simulink library "Traffic_2_UL"  (R2020a)
settings: Solver=VariableStepAuto  StartTime=0.0  StopTime=10.0  RelTol=1e-3
undefined symbols (not defined in the file): DiscIntNeverNeededParam, Int, sig_info, stopping_profile, T_mode, t_start, Traffic
libraries: simulink x8
settings Model: Creator=John Jr  LastModifiedBy=John Jr
settings DataIOCC: ReturnWorkspaceOutputs=off
settings DebuggingCC: ArithmeticOperatorsInVariantConditions=warning
settings SFSimCC: CustomCodeUndefinedFunction=UseInterfaceOnly

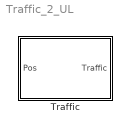
== system Traffic_2_UL ==
  Traffic : Subsystem
      mask Display:
      | patch([0 1 1 0], [0 0 1 1],[.8 1 1])
      | 
      | port_label('input',1,'Pos')
      | 
      | port_label('output',1,'Traffic')

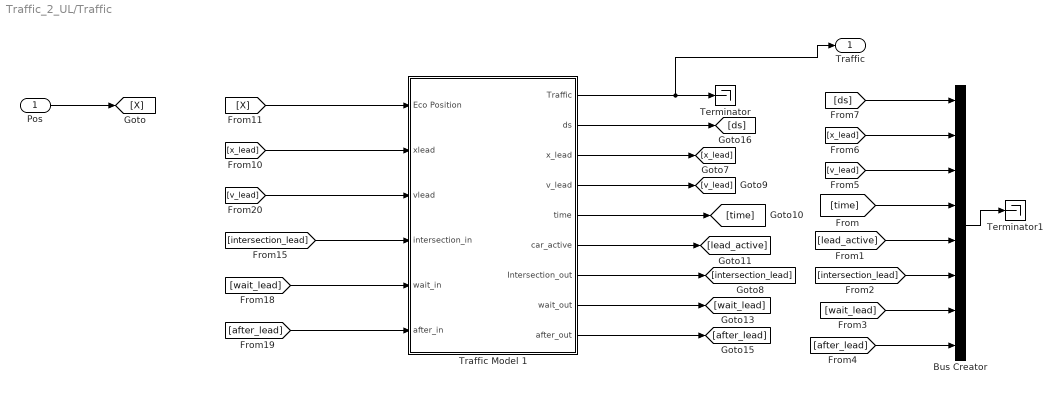
== system Traffic_2_UL/Traffic ==
  Pos : Inport
  Bus Creator : BusCreator  Inputs=8
  Terminator : Terminator
  Terminator1 : Terminator
  Traffic Model 1 : Subsystem
  Traffic : Outport  VectorParamsAs1DForOutWhenUnconnected=off
  wires:
  [ds] -> Bus Creator/1
  [x_lead] -> Bus Creator/2
  [v_lead] -> Bus Creator/3
  [time] -> Bus Creator/4
  [lead_active] -> Bus Creator/5
  [intersection_lead] -> Bus Creator/6
  [wait_lead] -> Bus Creator/7
  [after_lead] -> Bus Creator/8
  Traffic Model 1/3(x_lead) -> [x_lead]
  Traffic Model 1/6(car_active) -> [lead_active]
  [x_lead] -> Traffic Model 1/2(xlead)
  Traffic Model 1/4(v_lead) -> [v_lead]
  Traffic Model 1/9(after_out) -> [after_lead]
  [X] -> Traffic Model 1/1(Eco Position)
  Traffic Model 1/5(time) -> [time]
  Pos/1 -> [X]
  [after_lead] -> Traffic Model 1/6(after_in)
  Traffic Model 1/7(Intersection_out) -> [intersection_lead]
  [intersection_lead] -> Traffic Model 1/4(intersection_in)
  Traffic Model 1/2(ds) -> [ds]
  [v_lead] -> Traffic Model 1/3(vlead)
  Traffic Model 1/8(wait_out) -> [wait_lead]
  [wait_lead] -> Traffic Model 1/5(wait_in)
  Traffic Model 1/1(Traffic) -> Terminator/1, Traffic/1
  Bus Creator/1 -> Terminator1/1

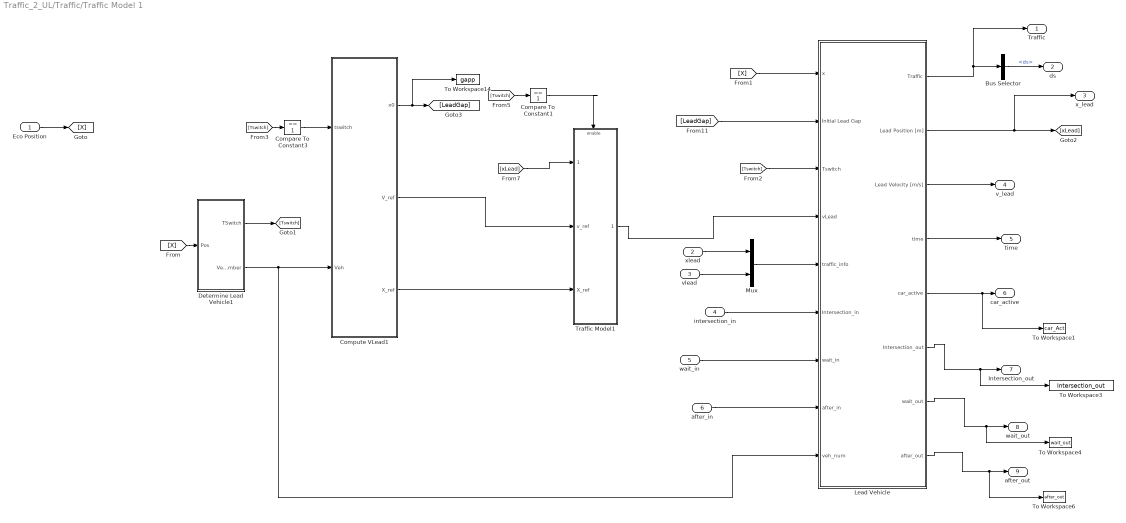
== system Traffic_2_UL/Traffic/Traffic Model 1 ==
  Eco Position : Inport
  xlead : Inport  Port=2
  vlead : Inport  Port=3
  intersection_in : Inport  Port=4
  wait_in : Inport  Port=5
  after_in : Inport  Port=6
  Bus Selector : BusSelector  OutputSignals=ds
  Compare To Constant1 : simulink/Logic and Bit Operations/Compare To Constant  relop===  const=1  OutDataTypeStr=boolean
  Compare To Constant3 : simulink/Logic and Bit Operations/Compare To Constant  relop===  const=1  OutDataTypeStr=boolean
  Compute VLead1 : Subsystem
  Determine Lead Vehicle1 : Subsystem
  Lead Vehicle : Subsystem
      settings: MinAlgLoopOccurrences=on
  Mux : Mux  Inputs=2
  To Workspace1 : ToWorkspace  VariableName=car_Act  SampleTime=.01
  To Workspace14 : ToWorkspace  VariableName=gapp  SampleTime=.01
  To Workspace3 : ToWorkspace  VariableName=Intersection_out  SampleTime=-1
  To Workspace4 : ToWorkspace  VariableName=wait_out  SampleTime=-1
  To Workspace6 : ToWorkspace  VariableName=after_out  SampleTime=-1
  Traffic Model1 : Subsystem
  Traffic : Outport  VectorParamsAs1DForOutWhenUnconnected=off
  ds : Outport  Port=2  VectorParamsAs1DForOutWhenUnconnected=off
  x_lead : Outport  Port=3  VectorParamsAs1DForOutWhenUnconnected=off
  v_lead : Outport  Port=4  VectorParamsAs1DForOutWhenUnconnected=off
  time : Outport  Port=5  VectorParamsAs1DForOutWhenUnconnected=off
  car_active : Outport  Port=6  VectorParamsAs1DForOutWhenUnconnected=off
  Intersection_out : Outport  Port=7  VectorParamsAs1DForOutWhenUnconnected=off
  wait_out : Outport  Port=8  VectorParamsAs1DForOutWhenUnconnected=off
  after_out : Outport  Port=9  VectorParamsAs1DForOutWhenUnconnected=off
  wires:
  Lead Vehicle/2(Lead Position [m]) -> [xLead], x_lead/1
  vlead/1 -> Mux/2
  [xLead] -> Traffic Model1/1(x_Lead)
  xlead/1 -> Mux/1
  Mux/1 -> Lead Vehicle/5(traffic_info)
  Bus Selector/1 -> ds/1  "<ds>"
  Traffic Model1/1(v_lead) -> Lead Vehicle/4(vLead)
  Compare To Constant1/1 -> Traffic Model1/Enable
  Determine Lead Vehicle1/2(Veh Number) -> Lead Vehicle/9(veh_num), Compute VLead1/2(Veh)
  intersection_in/1 -> Lead Vehicle/6(Intersection_in)
  wait_in/1 -> Lead Vehicle/7(wait_in)
  after_in/1 -> Lead Vehicle/8(after_in)
  Lead Vehicle/8(after_out) -> after_out/1, To Workspace6/1
  Lead Vehicle/7(wait_out) -> wait_out/1, To Workspace4/1
  Lead Vehicle/6(Intersection_out) -> Intersection_out/1, To Workspace3/1
  Lead Vehicle/5(car_active) -> car_active/1, To Workspace1/1
  Lead Vehicle/4(time) -> time/1
  Lead Vehicle/3(Lead Velocity [m/s]) -> v_lead/1
  Compute VLead1/3(X_ref) -> Traffic Model1/3(X_ref)
  Lead Vehicle/1(Traffic) -> Traffic/1, Bus Selector/1
  [Tswitch] -> Lead Vehicle/3(Tswitch)
  [X] -> Lead Vehicle/1(x)
  [LeadGap] -> Lead Vehicle/2(Initial Lead Gap)
  Compute VLead1/1(x0) -> [LeadGap], To Workspace14/1
  [Tswitch] -> Compare To Constant3/1
  Compute VLead1/2(V_ref) -> Traffic Model1/2(v_ref)
  Compare To Constant3/1 -> Compute VLead1/1(tswitch)
  [Tswitch] -> Compare To Constant1/1
  Determine Lead Vehicle1/1(TSwitch) -> [Tswitch]
  [X] -> Determine Lead Vehicle1/1(Pos)
  Eco Position/1 -> [X]

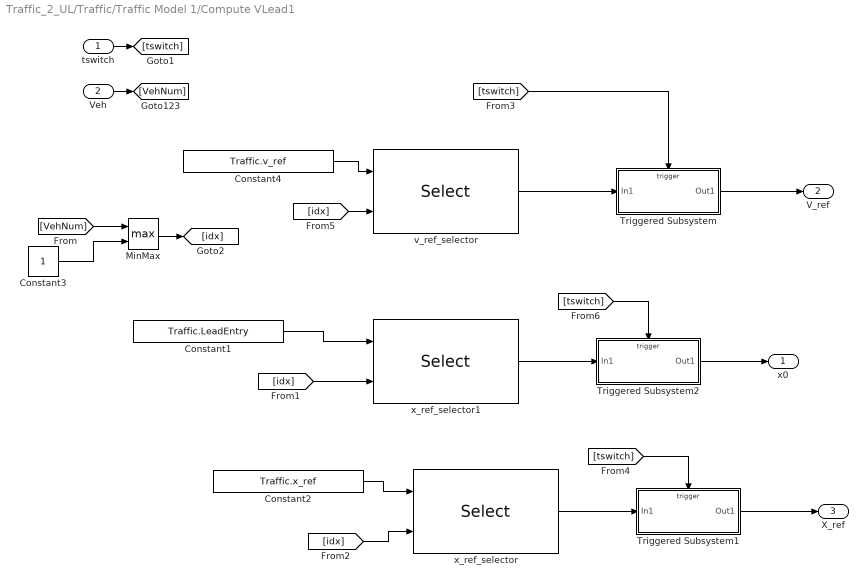
== system Traffic_2_UL/Traffic/Traffic Model 1/Compute VLead1 ==
  tswitch : Inport  PortDimensions=1
  Veh : Inport  Port=2  PortDimensions=1
  Constant1 : Constant  Value=Traffic.LeadEntry
  Constant2 : Constant  Value=Traffic.x_ref
  Constant3 : Constant
  Constant4 : Constant  Value=Traffic.v_ref
  MinMax : MinMax  Function=max  Inputs=2  InputSameDT=on
  Triggered Subsystem : Subsystem  TreatAsAtomicUnit=on
  Triggered Subsystem1 : Subsystem  TreatAsAtomicUnit=on
  Triggered Subsystem2 : Subsystem  TreatAsAtomicUnit=on
  v_ref_selector : Selector  NumberOfDimensions=2  InputPortWidth=3  IndexOptions=Select all,Index vector (port)  Indices=[1 3],1  OutputSizes=1,1
  x_ref_selector : Selector  NumberOfDimensions=2  InputPortWidth=3  IndexOptions=Select all,Index vector (port)  Indices=[1 3],1  OutputSizes=1,1
  x_ref_selector1 : Selector  InputPortWidth=40  IndexOptions=Index vector (port)  Indices=[1 3]  OutputSizes=1
  x0 : Outport  PortDimensions=1  VectorParamsAs1DForOutWhenUnconnected=off
  V_ref : Outport  Port=2  PortDimensions=[8000 1]  InitialOutput=ones(8000,1)  VectorParamsAs1DForOutWhenUnconnected=off
  X_ref : Outport  Port=3  PortDimensions=[8000 1]  VectorParamsAs1DForOutWhenUnconnected=off
  wires:
  [tswitch] -> Triggered Subsystem2/Trigger
  Triggered Subsystem2/1(Out1) -> x0/1
  x_ref_selector1/1 -> Triggered Subsystem2/1(In1)
  [idx] -> v_ref_selector/2
  [idx] -> x_ref_selector1/2
  Constant1/1 -> x_ref_selector1/1
  [tswitch] -> Triggered Subsystem1/Trigger
  Triggered Subsystem1/1(Out1) -> X_ref/1
  x_ref_selector/1 -> Triggered Subsystem1/1(In1)
  [idx] -> x_ref_selector/2
  MinMax/1 -> [idx]
  [tswitch] -> Triggered Subsystem/Trigger
  Triggered Subsystem/1(Out1) -> V_ref/1
  v_ref_selector/1 -> Triggered Subsystem/1(In1)
  tswitch/1 -> [tswitch]
  Constant3/1 -> MinMax/2
  [VehNum] -> MinMax/1
  Constant4/1 -> v_ref_selector/1
  Constant2/1 -> x_ref_selector/1
  Veh/1 -> [VehNum]

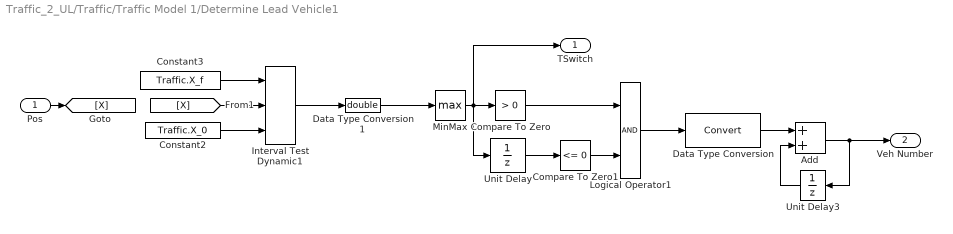
== system Traffic_2_UL/Traffic/Traffic Model 1/Determine Lead Vehicle1 ==
  Pos : Inport
  Add : Sum
  Compare To Zero : simulink/Logic and Bit Operations/Compare To Zero  relop=>  OutDataTypeStr=boolean
  Compare To Zero1 : simulink/Logic and Bit Operations/Compare To Zero  relop=<=  OutDataTypeStr=boolean
  Constant2 : Constant  Value=Traffic.X_0
  Constant3 : Constant  Value=Traffic.X_f
  Data Type Conversion : DataTypeConversion
  Data Type Conversion1 : DataTypeConversion  OutDataTypeStr=double
  Interval Test Dynamic1 : simulink/Logic and Bit Operations/Interval Test Dynamic  IntervalClosedRight=on  IntervalClosedLeft=on  OutDataTypeStr=boolean
      settings: SourceProductBaseCode=SL
  Logical Operator1 : Logic  OutDataTypeStr=boolean
  MinMax : MinMax  Function=max
  Unit Delay : UnitDelay  SampleTime=-1  HasFrameUpgradeWarning=on
  Unit Delay3 : UnitDelay  SampleTime=-1  HasFrameUpgradeWarning=on
  TSwitch : Outport  VectorParamsAs1DForOutWhenUnconnected=off
  Veh Number : Outport  Port=2  VectorParamsAs1DForOutWhenUnconnected=off
  wires:
  Pos/1 -> [X]
  [X] -> Interval Test Dynamic1/2
  Constant3/1 -> Interval Test Dynamic1/1
  Constant2/1 -> Interval Test Dynamic1/3
  Interval Test Dynamic1/1 -> Data Type Conversion1/1
  MinMax/1 -> TSwitch/1, Unit Delay/1, Compare To Zero/1
  Unit Delay/1 -> Compare To Zero1/1
  Compare To Zero1/1 -> Logical Operator1/2
  Compare To Zero/1 -> Logical Operator1/1
  Unit Delay3/1 -> Add/2
  Add/1 -> Veh Number/1, Unit Delay3/1
  Logical Operator1/1 -> Data Type Conversion/1
  Data Type Conversion/1 -> Add/1
  Data Type Conversion1/1 -> MinMax/1

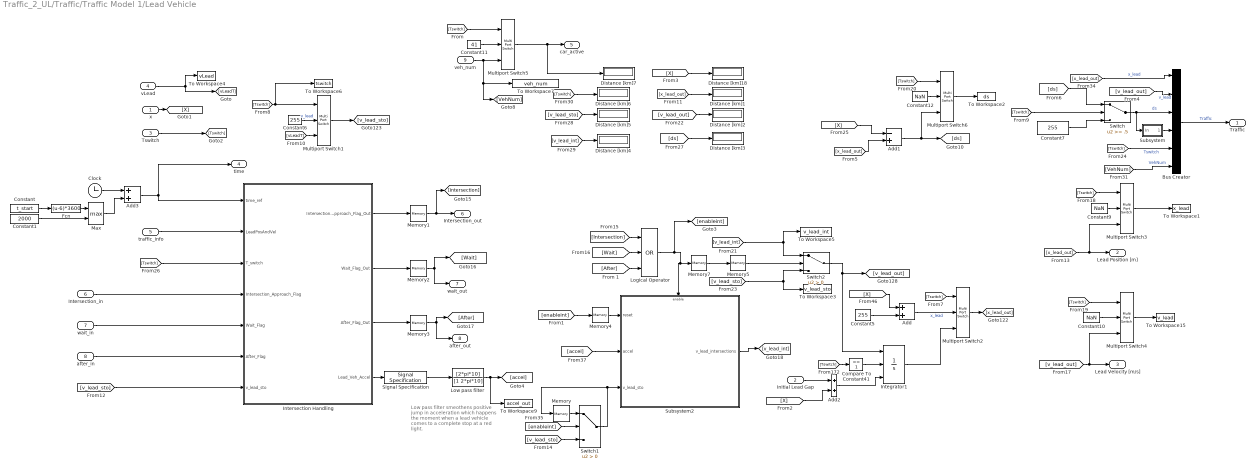
== system Traffic_2_UL/Traffic/Traffic Model 1/Lead Vehicle ==
  note: Low pass filter smeothens
      | positive jump in acceleration which
      | happens the moment when a lead
      | vehicle comes to a complete stop
      | at a red light.
  x : Inport
  Initial Lead Gap : Inport  Port=2
  Tswitch : Inport  Port=3
  vLead : Inport  Port=4
  traffic_info : Inport  Port=5
  Intersection_in : Inport  Port=6
  wait_in : Inport  Port=7
  after_in : Inport  Port=8
  veh_num : Inport  Port=9
  Add : Sum
  Add1 : Sum  Inputs=-+
  Add2 : Sum
  Add3 : Sum
  Bus Creator : BusCreator  Inputs=6
  Clock : Clock
      settings: Decimation=100
  Compare To Constant41 : simulink/Logic and Bit Operations/Compare To Constant  relop===  const=1  OutDataTypeStr=boolean
  Constant : Constant  Value=t_start
  Constant1 : Constant  Value=2000
  Constant10 : Constant  Value=NaN
  Constant11 : Constant  Value=41
  Constant12 : Constant  Value=NaN
  Constant5 : Constant  Value=255
  Constant6 : Constant  Value=255
  Constant7 : Constant  Value=255
  Constant9 : Constant  Value=NaN
  Distance [km]{1..7,18} (8 alike) : Display
      settings: Format=bank  Decimation=2
  Fcn : Fcn  Expr=(u-6)*3600
  Integrator1 : Integrator  ExternalReset=rising  InitialConditionSource=external  InitialCondition=2050  LimitOutput=on  LowerSaturationLimit=0
  Intersection Handling : Subsystem
  Logical Operator : Logic  Operator=OR  Inputs=3  AllPortsSameDT=off  OutDataTypeStr=boolean
  Low pass filter : TransferFcn  Numerator=[2*pi*10]  Denominator=[1 2*pi*10]
  Max : MinMax  Function=max  Inputs=2
  Memory{,1..5,7} (7 alike) : Memory
  Multiport Switch{1..6} (6 alike) : MultiPortSwitch  DataPortOrder=Zero-based contiguous  Inputs=2  DiagnosticForDefault=None  zeroidx=on
  Signal Specification : SignalSpecification  Dimensions=1
  Subsystem : Subsystem
  Subsystem2 : Subsystem
  Switch : Switch  Threshold=.5
  Switch1 : Switch  Criteria=u2 > Threshold
  Switch2 : Switch  Criteria=u2 > Threshold
  To Workspace1 : ToWorkspace  VariableName=x_lead  SampleTime=-1
  To Workspace15 : ToWorkspace  VariableName=v_lead  SampleTime=-1
  To Workspace2 : ToWorkspace  VariableName=ds  SampleTime=-1
  To Workspace3 : ToWorkspace  VariableName=v_lead_sto  SampleTime=-1
  To Workspace4 : ToWorkspace  VariableName=vLead  SampleTime=-1
  To Workspace5 : ToWorkspace  VariableName=v_lead_int  SampleTime=-1
  To Workspace6 : ToWorkspace  VariableName=tswitch  SampleTime=-1
  To Workspace7 : ToWorkspace  VariableName=veh_num  SampleTime=-1
  To Workspace9 : ToWorkspace  VariableName=accel_out  SampleTime=-1
  Traffic : Outport  VectorParamsAs1DForOutWhenUnconnected=off
  Lead Position [m] : Outport  Port=2  VectorParamsAs1DForOutWhenUnconnected=off
  Lead Velocity [m/s] : Outport  Port=3  VectorParamsAs1DForOutWhenUnconnected=off
  time : Outport  Port=4  VectorParamsAs1DForOutWhenUnconnected=off
  car_active : Outport  Port=5  VectorParamsAs1DForOutWhenUnconnected=off
  Intersection_out : Outport  Port=6  VectorParamsAs1DForOutWhenUnconnected=off
  wait_out : Outport  Port=7  VectorParamsAs1DForOutWhenUnconnected=off
  after_out : Outport  Port=8  VectorParamsAs1DForOutWhenUnconnected=off
  wires:
  Memory5/1 -> Switch2/2
  Memory4/1 -> Subsystem2/1("reset ")
  [enableint] -> Memory4/1
  Memory7/1 -> Memory5/1
  [v_lead_sto] -> Switch1/3
  [enableint] -> Switch1/2
  Memory/1 -> Switch1/1
  Low pass filter/1 -> [accel], To Workspace9/1
  Signal Specification/1 -> Low pass filter/1
  Switch1/1 -> Subsystem2/3("v_lead_sto "), Memory/1
  Intersection Handling/4(Lead_Veh_Accel) -> Signal Specification/1
  [Tswitch] -> Distance [km]6/1
  [v_lead_sto] -> Distance [km]5/1
  [v_lead_int] -> Distance [km]4/1
  [ds] -> Distance [km]3/1
  [v_lead_out] -> Distance [km]2/1
  [x_lead_out] -> Distance [km]1/1
  [X] -> Distance [km]18/1
  Memory3/1 -> after_out/1, [After]
  Memory2/1 -> [Wait], wait_out/1
  Memory1/1 -> Intersection_out/1, [Intersection]
  Intersection Handling/2(Wait_Flag_Out) -> Memory2/1
  Intersection Handling/3(After_Flag_Out) -> Memory3/1
  [Intersection] -> Logical Operator/1
  [Wait] -> Logical Operator/2
  [After] -> Logical Operator/3
  [v_lead_sto] -> Intersection Handling/7(v_lead_sto)
  after_in/1 -> Intersection Handling/6(After_Flag)
  wait_in/1 -> Intersection Handling/5(Wait_Flag)
  Intersection_in/1 -> Intersection Handling/4(Intersection_Approach_Flag)
  [Tswitch] -> Intersection Handling/3(T_switch)
  traffic_info/1 -> Intersection Handling/2(LeadPosAndVel)
  Intersection Handling/1("Intersection_Approach_Flag_Out ") -> Memory1/1
  Add3/1 -> time/1, Intersection Handling/1(time_ref)
  Multiport Switch6/1 -> To Workspace2/1
  Constant12/1 -> Multiport Switch6/2
  Add1/1 -> [ds], Multiport Switch6/3
  [Tswitch] -> Multiport Switch6/1
  Multiport Switch4/1 -> To Workspace15/1
  Constant10/1 -> Multiport Switch4/2
  [v_lead_out] -> Lead Velocity [m/s]/1, Multiport Switch4/3
  [Tswitch] -> Multiport Switch4/1
  Multiport Switch3/1 -> To Workspace1/1
  [Tswitch] -> Multiport Switch3/1
  Constant9/1 -> Multiport Switch3/2
  [x_lead_out] -> Lead Position [m]/1, Multiport Switch3/3
  Switch2/1 -> [v_lead_out], Integrator1/1
  Subsystem2/1(v_lead_intersections) -> [v_lead_int]
  Logical Operator/1 -> Memory7/1, Subsystem2/Enable, [enableint]
  [v_lead_sto] -> To Workspace3/1, Switch2/3
  [v_lead_int] -> Switch2/1, To Workspace5/1
  [accel] -> Subsystem2/2(accel)
  Constant5/1 -> Add/2
  [X] -> Add/1
  [x_lead_out] -> Add1/2
  [X] -> Add1/1
  Tswitch/1 -> [Tswitch]
  Constant11/1 -> Multiport Switch5/2
  veh_num/1 -> Multiport Switch5/3, To Workspace7/1, [VehNum]
  Multiport Switch5/1 -> car_active/1, Distance [km]7/1
  [Tswitch] -> Multiport Switch5/1
  Bus Creator/1 -> Traffic/1  "Traffic"
  x/1 -> [X]
  [vLeadT] -> Multiport Switch1/3
  Constant6/1 -> Multiport Switch1/2  "v_lead"
  Multiport Switch1/1 -> [v_lead_sto]
  [Tswitch] -> Multiport Switch1/1, To Workspace6/1
  Integrator1/1 -> Multiport Switch2/3
  [Tswitch] -> Multiport Switch2/1
  Add/1 -> Multiport Switch2/2  "x_lead"
  [Tswitch] -> Compare To Constant41/1
  Multiport Switch2/1 -> [x_lead_out]
  [X] -> Add2/2
  Add2/1 -> Integrator1/3
  Compare To Constant41/1 -> Integrator1/2
  vLead/1 -> [vLeadT], To Workspace4/1
  Initial Lead Gap/1 -> Add2/1
  [x_lead_out] -> Bus Creator/1  "x_lead"
  Subsystem/1(out) -> Bus Creator/4
  [Tswitch] -> Bus Creator/5  "Tswitch"
  Switch/1 -> Subsystem/1(In), Bus Creator/3  "ds"
  [ds] -> Switch/1
  [v_lead_out] -> Bus Creator/2  "v_lead"
  [VehNum] -> Bus Creator/6  "VehNum"
  Constant7/1 -> Switch/3
  [Tswitch] -> Switch/2
  Constant/1 -> Fcn/1
  Clock/1 -> Add3/1
  Fcn/1 -> Max/1
  Constant1/1 -> Max/2
  Max/1 -> Add3/2

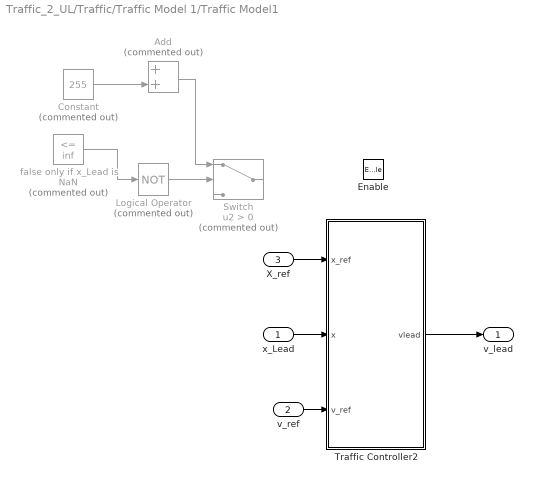
== system Traffic_2_UL/Traffic/Traffic Model 1/Traffic Model1 ==
  x_Lead : Inport
  v_ref : Inport  Port=2
  X_ref : Inport  Port=3
  Enable : EnablePort
  Add : Sum  Commented=on
  Constant : Constant  Commented=on  Value=255
  Logical Operator : Logic  Commented=on  Operator=NOT  AllPortsSameDT=off  OutDataTypeStr=boolean
  Switch : Switch  Commented=on  Criteria=u2 > Threshold
  Traffic Controller2 : MATLAB Function  TreatAsAtomicUnit=on
  false only if x_Lead is NaN : simulink/Logic and Bit Operations/Compare To Constant  Commented=on  relop=<=  const=inf  OutDataTypeStr=boolean
  v_lead : Outport  VectorParamsAs1DForOutWhenUnconnected=off
  wires:
  x_Lead/1 -> Traffic Controller2/2(x)
  Add/1 -> Switch/1
  Logical Operator/1 -> Switch/2
  Constant/1 -> Add/2
  false only if x_Lead is NaN/1 -> Logical Operator/1
  Traffic Controller2/1(vlead) -> v_lead/1
  v_ref/1 -> Traffic Controller2/3(v_ref)
  X_ref/1 -> Traffic Controller2/1(x_ref)

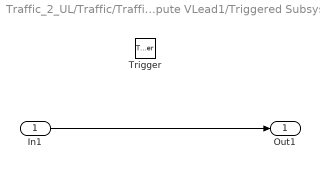
== system Traffic_2_UL/Traffic/Traffic Model 1/Compute VLead1/Triggered Subsystem ==
  In1 : Inport  PortDimensions=[8000 1]
  Trigger : TriggerPort  VariantControl=Variant
  Out1 : Outport  VectorParamsAs1DForOutWhenUnconnected=off
  wires:
  In1/1 -> Out1/1

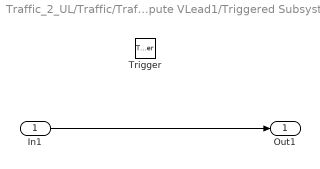
== system Traffic_2_UL/Traffic/Traffic Model 1/Compute VLead1/Triggered Subsystem1 ==
  In1 : Inport  PortDimensions=[8000 1]
  Trigger : TriggerPort  VariantControl=Variant
  Out1 : Outport  VectorParamsAs1DForOutWhenUnconnected=off
  wires:
  In1/1 -> Out1/1

== system Traffic_2_UL/Traffic/Traffic Model 1/Compute VLead1/Triggered Subsystem2 ==
  In1 : Inport  PortDimensions=1
  Trigger : TriggerPort  VariantControl=Variant
  Out1 : Outport  VectorParamsAs1DForOutWhenUnconnected=off
  wires:
  In1/1 -> Out1/1

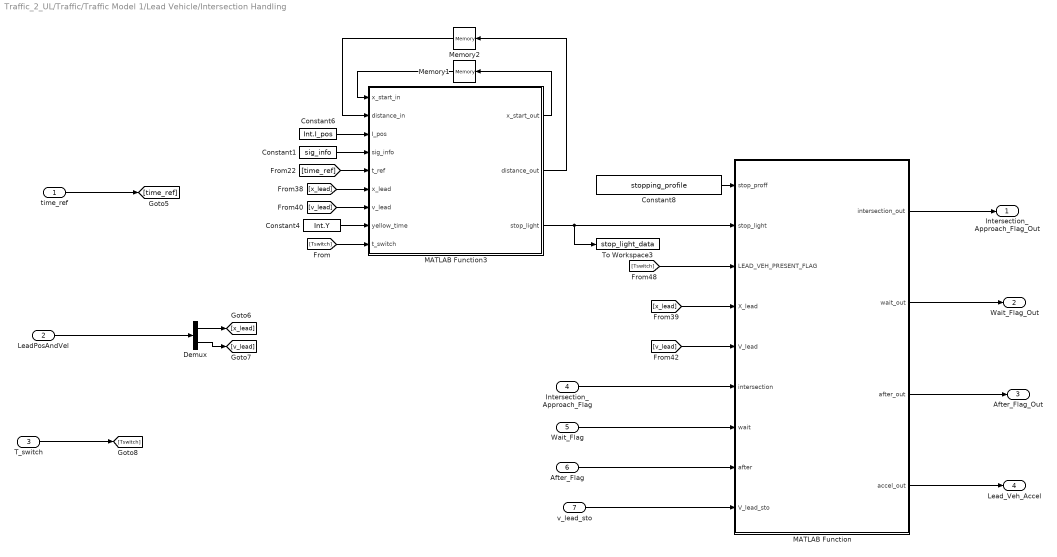
== system Traffic_2_UL/Traffic/Traffic Model 1/Lead Vehicle/Intersection Handling ==
  time_ref : Inport
  LeadPosAndVel : Inport  Port=2
  T_switch : Inport  Port=3
  Intersection_Approach_Flag : Inport  Port=4
  Wait_Flag : Inport  Port=5
  After_Flag : Inport  Port=6
  v_lead_sto : Inport  Port=7
  Constant1 : Constant  Value=sig_info
  Constant4 : Constant  Value=Int.Y
  Constant6 : Constant  Value=Int.I_pos
  Constant8 : Constant  Value=stopping_profile
  Demux : Demux  Outputs=2
  MATLAB Function : MATLAB Function  TreatAsAtomicUnit=on
  MATLAB Function3 : MATLAB Function  TreatAsAtomicUnit=on
  Memory1 : Memory
  Memory2 : Memory
  To Workspace3 : ToWorkspace  VariableName=stop_light_data  SampleTime=-1
  "Intersection_Approach_Flag_Out " : Outport  VectorParamsAs1DForOutWhenUnconnected=off
  Wait_Flag_Out : Outport  Port=2  VectorParamsAs1DForOutWhenUnconnected=off
  After_Flag_Out : Outport  Port=3  VectorParamsAs1DForOutWhenUnconnected=off
  Lead_Veh_Accel : Outport  Port=4  VectorParamsAs1DForOutWhenUnconnected=off
  wires:
  LeadPosAndVel/1 -> Demux/1
  [Tswitch] -> MATLAB Function3/9(t_switch)
  T_switch/1 -> [Tswitch]
  [time_ref] -> MATLAB Function3/5(t_ref)
  v_lead_sto/1 -> MATLAB Function/9(V_lead_sto)
  time_ref/1 -> [time_ref]
  [x_lead] -> MATLAB Function3/6(x_lead)
  [v_lead] -> MATLAB Function3/7(v_lead)
  Demux/2 -> [v_lead]
  Demux/1 -> [x_lead]
  [v_lead] -> MATLAB Function/5(V_lead)
  [x_lead] -> MATLAB Function/4(X_lead)
  [Tswitch] -> MATLAB Function/3(LEAD_VEH_PRESENT_FLAG)
  MATLAB Function/4(accel_out) -> Lead_Veh_Accel/1
  Wait_Flag/1 -> MATLAB Function/7(wait)
  After_Flag/1 -> MATLAB Function/8(after)
  MATLAB Function3/3(stop_light) -> MATLAB Function/2(stop_light), To Workspace3/1
  MATLAB Function3/1(x_start_out) -> Memory1/1
  MATLAB Function3/2(distance_out) -> Memory2/1
  MATLAB Function/1(intersection_out) -> "Intersection_Approach_Flag_Out "/1
  MATLAB Function/2(wait_out) -> Wait_Flag_Out/1
  Constant4/1 -> MATLAB Function3/8(yellow_time)
  Constant6/1 -> MATLAB Function3/3(I_pos)
  MATLAB Function/3(after_out) -> After_Flag_Out/1
  Intersection_Approach_Flag/1 -> MATLAB Function/6(intersection)
  Memory1/1 -> MATLAB Function3/1(x_start_in)
  Constant8/1 -> MATLAB Function/1(stop_proff)
  Memory2/1 -> MATLAB Function3/2(distance_in)
  Constant1/1 -> MATLAB Function3/4(sig_info)

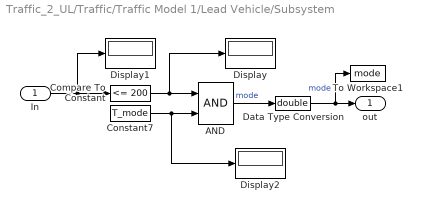
== system Traffic_2_UL/Traffic/Traffic Model 1/Lead Vehicle/Subsystem ==
  In : Inport
  AND : Logic  IconShape=distinctive  AllPortsSameDT=off  OutDataTypeStr=boolean
  Compare To Constant : simulink/Logic and Bit Operations/Compare To Constant  relop=<=  const=200  OutDataTypeStr=boolean
  Constant7 : Constant  Value=T_mode
  Data Type Conversion : DataTypeConversion  OutDataTypeStr=double
  Display : Display
  Display1 : Display
  Display2 : Display
  To Workspace1 : ToWorkspace  VariableName=mode  SampleTime=-1
  out : Outport  VectorParamsAs1DForOutWhenUnconnected=off
  wires:
  Constant7/1 -> Display2/1, AND/2
  Compare To Constant/1 -> Display/1, AND/1
  In/1 -> Display1/1, Compare To Constant/1
  AND/1 -> Data Type Conversion/1  "mode"
  Data Type Conversion/1 -> To Workspace1/1, out/1  "mode"

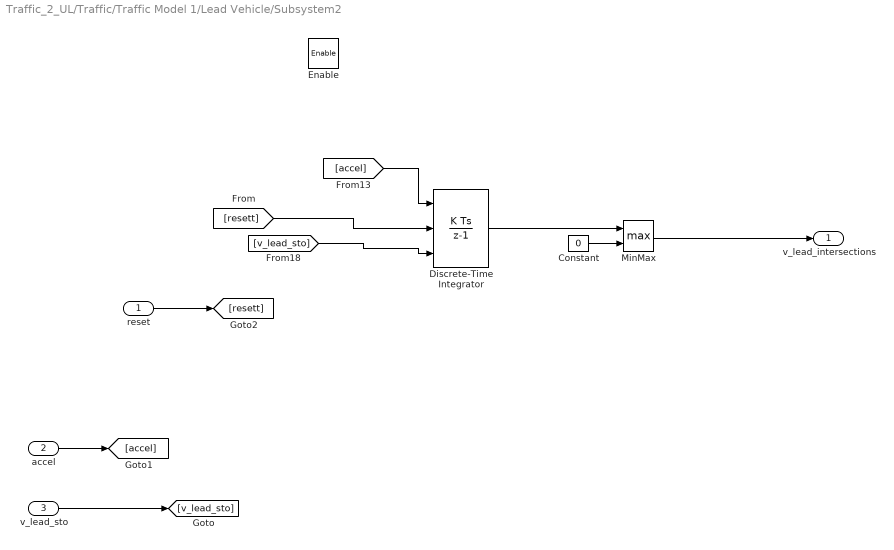
== system Traffic_2_UL/Traffic/Traffic Model 1/Lead Vehicle/Subsystem2 ==
  "reset " : Inport
  accel : Inport  Port=2
  "v_lead_sto " : Inport  Port=3
  Enable : EnablePort
  Constant : Constant  Value=0
  Discrete-Time Integrator : DiscreteIntegrator  ExternalReset=rising  InitialConditionSource=external  SampleTime=-1  ICPrevOutput=DiscIntNeverNeededParam  ICPrevScaledInput=DiscIntNeverNeededParam
  MinMax : MinMax  Function=max  Inputs=2
  v_lead_intersections : Outport  VectorParamsAs1DForOutWhenUnconnected=off
  wires:
  [resett] -> Discrete-Time Integrator/2
  "reset "/1 -> [resett]
  Constant/1 -> MinMax/2
  MinMax/1 -> v_lead_intersections/1
  "v_lead_sto "/1 -> [v_lead_sto]
  accel/1 -> [accel]
  [accel] -> Discrete-Time Integrator/1
  Discrete-Time Integrator/1 -> MinMax/1
  [v_lead_sto] -> Discrete-Time Integrator/3

== matlab function Traffic_2_UL/Traffic/Traffic Model 1/Lead Vehicle/Intersection Handling/MATLAB Function ==
  data: stop_proff input; stop_light input; LEAD_VEH_PRESENT_FLAG input; X_lead input; V_lead input; intersection input; wait input; after input; V_lead_sto input; intersection_out output; wait_out output; after_out output; accel_out output
function [intersection_out, wait_out, after_out,...
      accel_out] = intersection_sim(stop_proff, stop_light,...
      LEAD_VEH_PRESENT_FLAG, X_lead,V_lead, intersection, wait, after,...
      V_lead_sto)
% https://www.sciencedirect.com/science/article/pii/S1474667016442102   [1]
% http://ieeexplore.ieee.org/stamp/stamp.jsp?tp=&arnumber=6214590       [2]
lookahead_distance = 200;
stopping_profile = stop_proff;
buffer = 5;

if LEAD_VEH_PRESENT_FLAG == 0
    accel_out = 0;
    intersection_out = 0;
    wait_out = 0;
    after_out = 0;

else

    stop_location = stop_light(1);
    if intersection == 1   %Intersection flag has already been initialted
    %% approaching intersection
        if stop_location == 0 %light turns green during intersection approach phase
            after_out = 1;
            wait_out = 0;
            intersection_out = 0;
            accel_out = 0;
        else
            a_bstar = stopping_profile(3,:);
            x_bstar = stopping_profile(1,:);
            v_bstar = stopping_profile(2,:);
            X_q = -X_lead + (stop_location - buffer);
            v_bstar_val = interpone(x_bstar, v_bstar, X_q, 'str', 0);
            a_bstar_val = interpone(x_bstar, a_bstar, X_q, 'str', 0);
            accel = a_bstar_val*(V_lead/v_bstar_val)^2;       %   equation 9 of paper [2]

            if stop_location - X_lead < 0.02  %need to add a case for when if v_lead <0.1ms stop
                accel_out = 0;
                intersection_out = 0;
                wait_out = 1;
                after_out = 0;
            else
                accel_out = accel;
                intersection_out = 1;
                wait_out = 0;
                after_out = 0;
            end
        end
    elseif wait == 1   % wait_outing for light to turn green
    %% stopped at light
        if stop_location == 0 %  light turns green
            after_out = 1;
            wait_out = 0;
            intersection_out = 0;
            accel_out = 1;
        else
            accel_out = 1;
            intersection_out = 0;
            wait_out = 1;
            after_out = 0;
        end
    elseif after == 1       %   light has turned green
        %% leaving light after slowing down or stopping (intersection case entered beforehand)
        if V_lead_sto - V_lead <= 0.1 && V_lead_sto - V_lead >= -0.1 %reaches stochastic velocity
            intersection_out = 0;
            wait_out = 0;
            after_out = 0;
            accel_out = 0; % m/s^2
        elseif stop_location - X_lead < min(60*V_lead, lookahead_distance) && stop_location - X_lead > 0 %another intersection appears while accelerating to stochastic velocity profile.
            accel_out = 0;
            intersection_out = 1;
            wait_out = 0;
            after_out = 0;
        elseif V_lead_sto - V_lead > 0.1
            accel_out = 1; % m/s^2
            intersection_out = 0;
            wait_out = 0;
            after_out = 1;
        else
            accel_out = -1; % m/s^2   shouldn't happen
            intersection_out = 0;
            wait_out = 0;
            after_out = 1;
        end
    else
        if stop_location - X_lead < lookahead_distance && stop_location - X_lead > 0
            intersection_out = 1;
            wait_out = 0;
            after_out = 0;
            accel_out = 0;
        else
            accel_out = 0;
            intersection_out = 0;
            wait_out = 0;
            after_out = 0;
        end
    end
end
end
function return_val = interpone(X_data, Y_data, X_q, str, extrapval)
    if X_q >= X_data(1) && X_q <= X_data(end) 
        [~, I] = min((X_q - X_data).^2);
        if X_data(I) > X_q
            x_ub = X_data(I);
            x_lb = X_data(I-1);
            ind_xub = I;
            ind_xlb = I-1;
        else
            x_lb = X_data(I);
            ind_xlb = I;
            if I+1 >= length(X_data)    % M is probably equal to X_q and also the max value 
                x_lb = X_data(I-1);
                x_ub = I;
                ind_xub = I;
                ind_xlb = I-1;
            else
                x_ub = X_data(I+1);
                ind_xub = I+1;
            end
        end 
        y_0 = Y_data(ind_xlb);
        y_1 = Y_data(ind_xub);
        return_val = y_0 + (X_q - x_lb)*((y_1 - y_0)/(x_ub - x_lb));  
    elseif X_q <= X_data(1) && X_q >= X_data(end) 
        [~, I] = min((X_q - X_data).^2);
        if X_data(I) > X_q
            x_ub = X_data(I);
            ind_xub = I;
%             if I+1 >= length(X_data)    % M is probably equal to X_q and also the min value
%                 x_lb = X_data(I-1);
%                 x_ub = I;
%                 ind_xub = I;
%                 ind_xlb = I-1;
%             else
                x_lb = X_data(I+1);
                ind_xlb = I+1;
%             end
        else
            x_lb = X_data(I);
            ind_xlb = I;
            x_ub = X_data(I-1);
            ind_xub = I-1;
        end
        y_0 = Y_data(ind_xlb);
        y_1 = Y_data(ind_xub);
        return_val = y_0 + (X_q - x_lb)*((y_1 - y_0)/(x_ub - x_lb));  
    else 
        return_val = extrapval;
    end
end

== matlab function Traffic_2_UL/Traffic/Traffic Model 1/Lead Vehicle/Intersection Handling/MATLAB Function3 ==
  data: x_start_in input; distance_in input; x_start_out output; distance_out output; I_pos input; sig_info input; stop_light output; t_ref input; x_lead input; v_lead input; yellow_time input; t_switch input
function [x_start_out, distance_out, stop_light] = beat_the_light_question_mark(x_start_in, distance_in, I_pos,sig_info, t_ref, x_lead, v_lead, yellow_time, t_switch)
% stop_light is 3x1 arry containing the location, t_green, t_red of the
% upcoming stoplight
G = sig_info(:,:,2);                                    %   s - Intersection green phases 
Cs = sig_info(:,:,3);                                   %   s - Cycle start times 
C = sig_info(:,:,1);                                   %   s - Cycle start times 
lookahead_distance = 150;
buffer = 0;
if t_switch == 0 || isnan(I_pos(1))
    stop_light = [0; 0; 0];
    x_start_out = 0;
    distance_out = 0;
else
    diff = I_pos - x_lead;
    d = diff >= 0;
    [~, J] = max(d);
    ind = J(1);
    %find out if light is green
    ind2 = find(Cs(ind,:) <= t_ref,1,'last');         %   Current cycle # for upcoming intersection
    t_green = G(ind,ind2(1));
    t_light = C(ind,ind2(1));
    t_red = t_light - t_green;
    rem = t_ref-Cs(ind,ind2(1));
    stop_location = I_pos(ind,1);
    if max(I_pos(:,1)) - x_lead < 0
        stop_light = [0; 0; 0];  %your past the light   
        x_start_out = 0;
        distance_out = 0;
    elseif rem > t_green - yellow_time(ind) && stop_location - x_lead < lookahead_distance%light turns red, treating the last 6 seconds of t_green as a yellow light
        distance_to_make_light = yellow_time(ind)*v_lead;
        if x_start_in == 0
           x_start_out = x_lead; 
           x_start_in = x_lead;
           distance_out = distance_to_make_light;  
           distance_in = distance_to_make_light;
        end
        if stop_location - x_start_in < distance_in
            stop_light = [0; 0; 0];  %it's safe to run yellow
            x_start_out = x_start_in;
            distance_out = distance_in;
        else
            stop_light = [stop_location - buffer; t_green; t_red];
            x_start_out = x_start_in;
            distance_out = distance_in;
        end
    else %currently a green light
        stop_light = [0; 0; 0];  %essentially removes stoplight from road
        x_start_out = 0;
        distance_out = 0;
    end
    
end


%outputs zero if we make the green light

== matlab function Traffic_2_UL/Traffic/Traffic Model 1/Traffic Model1/Traffic Controller2 ==
  data: x_ref input; x input; v_ref input; vlead output size=1
function vlead = fcn(x_ref,x, v_ref)
    [a,~] = find(min(abs(x_ref-x))==abs(x_ref-x));
    if x_ref(a) == x
        vlead = v_ref(a(1));
    elseif x_ref(a) < x
        b = a(1)+1;
        y1 = (x-x_ref(a))/(x_ref(b)-x_ref(a(1)));
        y2 = (x_ref(b)-x)/(x_ref(b)-x_ref(a(1)));
        vlead = v_ref(a(1))*y2(1)+v_ref(b(1))*y1(1);
    else
        b = a(1)-1;
        y1 = (x-x_ref(b))/(x_ref(a(1))-x_ref(b));
        y2 = (x_ref(a(1))-x)/(x_ref(a(1))-x_ref(b));
        vlead = v_ref(b(1))*y2+v_ref(a(1))*y1;
    end
end
